simulink model "motor_control"  (R2023b)
settings: Solver=VariableStepAuto  StartTime=0.0  StopTime=10.0  RelTol=1e-3
values from neighbouring files (symbols this model uses):
  K = 1.8    [run_motor_control.m]    (also in run_motor_sim.m)
  Kp = 10    [run_motor_control.m]
  sigma = 16    [run_motor_control.m]    (also in run_motor_sim.m)
libraries: simulink x1
settings Model: Creator=Luca Ciancanelli  LastModifiedBy=Luca Ciancanelli

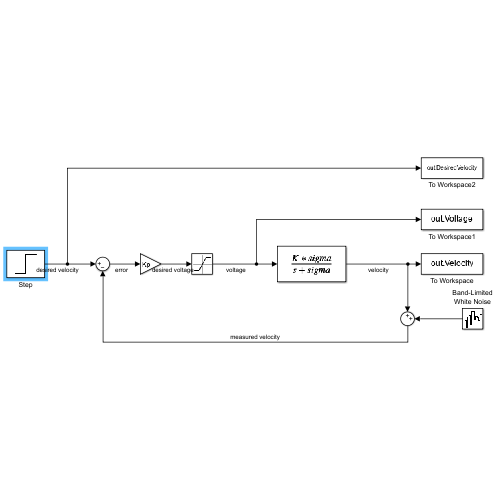
[thumbnail: Simulink's stored preview of the top-level diagram]
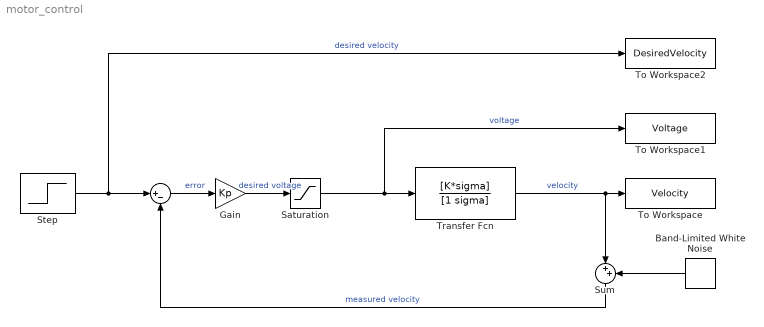
== system motor_control ==
  "    " : Sum  Inputs=|+-
  Band-Limited White Noise : simulink/Sources/Band-Limited White Noise  Cov=[0.0001]  Ts=0.01  seed=[23341]
  Gain : Gain  Gain=Kp
  Saturation : Saturate  UpperLimit=7.5  LowerLimit=-7.5
  Step : Step  After=3  SampleTime=0
  Sum : Sum  Inputs=|++
  To Workspace : ToWorkspace  VariableName=Velocity  SaveFormat=Timeseries  SampleTime=-1
  To Workspace1 : ToWorkspace  VariableName=Voltage  SaveFormat=Timeseries  SampleTime=-1
  To Workspace2 : ToWorkspace  VariableName=DesiredVelocity  SaveFormat=Timeseries  SampleTime=-1
  Transfer Fcn : TransferFcn  Numerator=[K*sigma]  Denominator=[1 sigma]
  wires:
  Transfer Fcn/1 -> Sum/1, To Workspace/1  "velocity"
  Step/1 -> To Workspace2/1, "    "/1  "desired velocity"
  "    "/1 -> Gain/1  "error"
  Gain/1 -> Saturation/1  "desired voltage"
  Saturation/1 -> To Workspace1/1, Transfer Fcn/1  "voltage"
  Band-Limited White Noise/1 -> Sum/2
  Sum/1 -> "    "/2  "measured velocity"
